simulink model "Mass_spring_dumber"  (R2022b)
settings: Solver=VariableStepAuto  StartTime=0.0  StopTime=10.0  FixedStep=1e-3  MaxStep=1e-3  RelTol=1e-3
values from neighbouring files (symbols this model uses):
  b = 10    [script_mass_damber.m]
  k = 400    [script_mass_damber.m]
  m = massvalue(i)    [script_mass_damber.m]
  x = 1    [script_mass_damber.m]
settings Model: Creator=Abanob_Sameh  LastModifiedBy=Abanob_Sameh
settings DataIOCC: SaveFormat=Structure

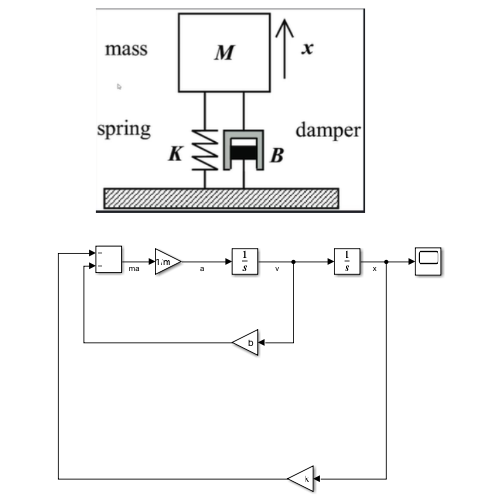
[thumbnail: Simulink's stored preview of the top-level diagram]
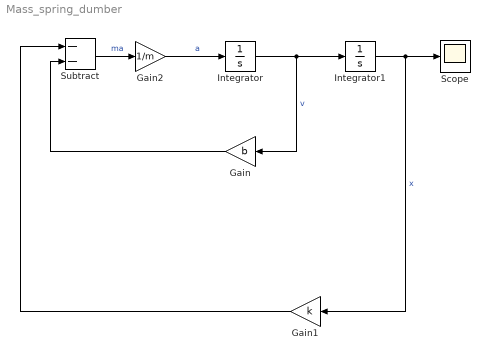
== system Mass_spring_dumber ==
  Gain : Gain  Gain=b
  Gain1 : Gain  Gain=k
  Gain2 : Gain  Gain=1/m
  Integrator : Integrator
  Integrator1 : Integrator  InitialCondition=x
  Scope : Scope
  Subtract : Sum  Inputs=--
  wires:
  Integrator/1 -> Gain/1, Integrator1/1  "v"
  Gain2/1 -> Integrator/1  "a"
  Integrator1/1 -> Gain1/1, Scope/1  "x"
  Subtract/1 -> Gain2/1  "ma"
  Gain/1 -> Subtract/2
  Gain1/1 -> Subtract/1
